simulink model "SC_LQR_simple_voltage_model"  (R2023a)
settings: Solver=VariableStepAuto  StartTime=0.0  StopTime=200  RelTol=1e-3
values from neighbouring files (symbols this model uses):
  A_model = [A11 zeros(3) A13 ... (first row only)    [LQR_state_space.m]
  B_model = [I^-1 I^-1 I^-1 ... (first row only)    [LQR_state_space.m]
  C_model = [eye(3) zeros(3) zeros(3) ... (first row only)    [LQR_state_space.m]
  D_model = [zeros(3) zeros(3) zeros(3) ... (first row only)    [LQR_state_space.m]
  I = 1e-7*[336109.715 0 0 ... (first row only)    [LQR_state_space.m]
  K1 = K(1:3,:)    [LQR_state_space.m]
  K2 = K(4:6,:)    [LQR_state_space.m]
  K3 = K(7:9,:)    [LQR_state_space.m]
  x0 = zeros(9,1)    [LQR_state_space.m]
undefined symbols (not defined in the file or in its folder): A, A_motor, B, B_motor, C_motor, D_motor, J, juliandate, K, Ke, Kt, La, n_cal, R_mgt, Ra, T_ext, T_max, T_max_mgt
libraries: matrix_library x15, slpidlib x15, simulink_extras x6, sharedutil x3, aerolibutil x2, vrlib x2, aerolibcubesatveh x1, aerolibgravity2 x1
(part 2 of 3)

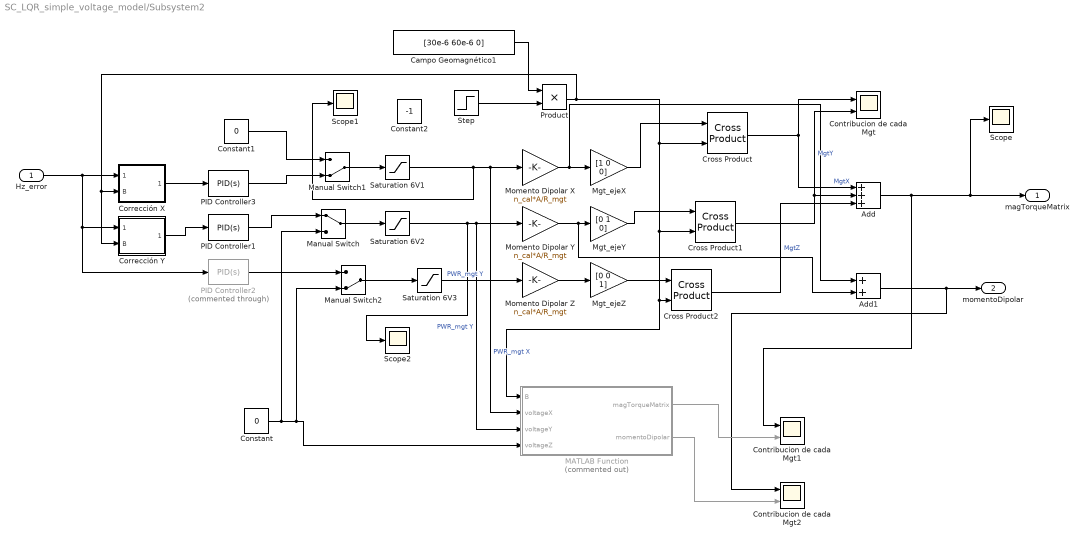
== system SC_LQR_simple_voltage_model/Subsystem2 ==
  Hz_error : Inport
  Add : Sum  Inputs=+++
  Add1 : Sum
  Campo Geomagnético1 : Constant  Value=[30e-6 60e-6 0]
  Constant : Constant  Value=0
  Constant1 : Constant  Value=0
  Constant2 : Constant  Value=-1
  Contribucion de cada Mgt : Scope  NumInputPorts=2
  Contribucion de cada Mgt1 : Scope  NumInputPorts=2
  Contribucion de cada Mgt2 : Scope  NumInputPorts=2
  Corrección X : MATLAB Function  TreatAsAtomicUnit=on
  Corrección Y : MATLAB Function  TreatAsAtomicUnit=on
  Cross Product : matrix_library/Cross Product
  Cross Product1 : matrix_library/Cross Product
  Cross Product2 : matrix_library/Cross Product
  MATLAB Function : MATLAB Function  Commented=on  TreatAsAtomicUnit=on
  Manual Switch : ManualSwitch
  Manual Switch1 : ManualSwitch  CurrentSetting=0
  Manual Switch2 : ManualSwitch  CurrentSetting=0
  Mgt_ejeX : Gain  Gain=[1 0 0]
  Mgt_ejeY : Gain  Gain=[0 1 0]
  Mgt_ejeZ : Gain  Gain=[0 0 1]
  Momento Dipolar X : Gain  Gain=n_cal*A/R_mgt
  Momento Dipolar Y : Gain  Gain=n_cal*A/R_mgt
  Momento Dipolar Z : Gain  Gain=n_cal*A/R_mgt
  PID Controller1 : slpidlib/PID Controller  Controller=PID  Form=Parallel  TimeDomain=Continuous-time  UseExternalTs=off  SampleTime=-1  IntegratorMethod=Forward Euler  FilterMethod=Forward Euler  ControllerParametersSource=internal  P=4500  I=800  UseKiTs=off  D=8000  N=100  UseFilter=on  TunerSelectOption=Transfer Function Based (PID Tuner App)  InitialConditionSource=internal  InitialConditionForIntegrator=0  InitialConditionForFilter=0  DifferentiatorICPrevScaledInput=0  ExternalReset=none  TrackingMode=off  Kt=1  LimitOutput=off  SatLimitsSource=internal  UpperSaturationLimit=1  LowerSaturationLimit=-1  LinearizeAsGain=on  AntiWindupMode=none  Kb=1  LimitIntegrator=off  UpperIntegratorSaturationLimit=inf  LowerIntegratorSaturationLimit=-inf  POutMin=[]  POutMax=[]  IOutMin=[]  IOutMax=[]  DOutMin=[]  DOutMax=[]  NOutMin=[]  NOutMax=[]  SumOutMin=[]  SumOutMax=[]  SaturationOutMin=[]  SaturationOutMax=[]  PParamMin=[]  PParamMax=[]  IParamMin=[]  IParamMax=[]  DParamMin=[]  DParamMax=[]  NParamMin=[]  NParamMax=[]  KbParamMin=[]  KbParamMax=[]  KtParamMin=[]  KtParamMax=[]  KbOutMin=[]  KbOutMax=[]  KtOutMin=[]  KtOutMax=[]  IntegratorOutMin=[]  IntegratorOutMax=[]  FilterOutMin=[]  FilterOutMax=[]  SumI1OutMin=[]  SumI1OutMax=[]  SumI2OutMin=[]  SumI2OutMax=[]  SumI3OutMin=[]  SumI3OutMax=[]  SumI4OutMin=[]  SumI4OutMax=[]  SumDOutMin=[]  SumDOutMax=[]  DifferentiatorOutMin=[]  DifferentiatorOutMax=[]  FilterDiffOutCoefMin=[]  FilterDiffOutCoefMax=[]  ReciprocalOutMin=[]  ReciprocalOutMax=[]  SumDenOutMin=[]  SumDenOutMax=[]  SumNumOutMin=[]  SumNumOutMax=[]  DivideOutMin=[]  DivideOutMax=[]  UdiffTsProdOutMin=[]  UdiffTsProdOutMax=[]  NTsProdOutMin=[]  NTsProdOutMax=[]  UintegralTsProdOutMin=[]  UintegralTsProdOutMax=[]  UngainTsProdOutMin=[]  UngainTsProdOutMax=[]  ClampingZeroOutDataTypeStr=Inherit: Inherit via back propagation  ClampingZeroOutMin=[]  ClampingZeroOutMax=[]  FilterDenConstantOutDataTypeStr=Inherit: Inherit via back propagation  FilterDenConstantOutMin=[]  FilterDenConstantOutMax=[]  PCopyOutDataTypeStr=Inherit: Inherit via back propagation  PCopyOutMin=[]  PCopyOutMax=[]  NCopyOutDataTypeStr=Inherit: Inherit via back propagation  NCopyOutMin=[]  NCopyOutMax=[]  IntegratorContinuousStateAttributes=''  IntegratorStateMustResolveToSignalObject=off  IntegratorRTWStateStorageClass=Auto  FilterContinuousStateAttributes=''  FilterStateMustResolveToSignalObject=off  FilterRTWStateStorageClass=Auto  ParallelPVariant=InternalParameters  IdealPVariant=Disabled  IVariant=InternalParameters  DVariant=InternalParameters  IntegratorVariant=Continuous  SatVariant=Disabled  AWVariant=Passthrough  PCopyVariant=Disabled  TRVariant=Disabled  FdbkBlocksVariant=Forward  IdealPFdbkVariant=Disabled  SatFdbkVariant=Disabled  DerivativeFilterVariant=ContFilter  NVariant=InternalParameters  NCopyVariant=Disabled  FilterICVariant=InternalICsFilter  IntegratorICVariant=InternalICs  ExternalResetVariant=Disabled  TRSumVariant=Passthrough  SumFdbkVariant=Disabled  SumVariant=Sum_PID  TsampFilterVariant=InternalTs  TsampNgainVariant=Passthrough  TsampIntegralVariant=Disabled_SignalSpec  ExternalSaturationOutDataTypeStr=Inherit: Same as second input
  PID Controller2 : slpidlib/PID Controller  Commented=through  Controller=PID  Form=Parallel  TimeDomain=Continuous-time  UseExternalTs=off  SampleTime=-1  IntegratorMethod=Forward Euler  FilterMethod=Forward Euler  ControllerParametersSource=internal  P=4500  I=800  UseKiTs=off  D=8000  N=100  UseFilter=on  TunerSelectOption=Transfer Function Based (PID Tuner App)  InitialConditionSource=internal  InitialConditionForIntegrator=0  InitialConditionForFilter=0  DifferentiatorICPrevScaledInput=0  ExternalReset=none  TrackingMode=off  Kt=1  LimitOutput=off  SatLimitsSource=internal  UpperSaturationLimit=1  LowerSaturationLimit=-1  LinearizeAsGain=on  AntiWindupMode=none  Kb=1  LimitIntegrator=off  UpperIntegratorSaturationLimit=inf  LowerIntegratorSaturationLimit=-inf  POutMin=[]  POutMax=[]  IOutMin=[]  IOutMax=[]  DOutMin=[]  DOutMax=[]  NOutMin=[]  NOutMax=[]  SumOutMin=[]  SumOutMax=[]  SaturationOutMin=[]  SaturationOutMax=[]  PParamMin=[]  PParamMax=[]  IParamMin=[]  IParamMax=[]  DParamMin=[]  DParamMax=[]  NParamMin=[]  NParamMax=[]  KbParamMin=[]  KbParamMax=[]  KtParamMin=[]  KtParamMax=[]  KbOutMin=[]  KbOutMax=[]  KtOutMin=[]  KtOutMax=[]  IntegratorOutMin=[]  IntegratorOutMax=[]  FilterOutMin=[]  FilterOutMax=[]  SumI1OutMin=[]  SumI1OutMax=[]  SumI2OutMin=[]  SumI2OutMax=[]  SumI3OutMin=[]  SumI3OutMax=[]  SumI4OutMin=[]  SumI4OutMax=[]  SumDOutMin=[]  SumDOutMax=[]  DifferentiatorOutMin=[]  DifferentiatorOutMax=[]  FilterDiffOutCoefMin=[]  FilterDiffOutCoefMax=[]  ReciprocalOutMin=[]  ReciprocalOutMax=[]  SumDenOutMin=[]  SumDenOutMax=[]  SumNumOutMin=[]  SumNumOutMax=[]  DivideOutMin=[]  DivideOutMax=[]  UdiffTsProdOutMin=[]  UdiffTsProdOutMax=[]  NTsProdOutMin=[]  NTsProdOutMax=[]  UintegralTsProdOutMin=[]  UintegralTsProdOutMax=[]  UngainTsProdOutMin=[]  UngainTsProdOutMax=[]  ClampingZeroOutDataTypeStr=Inherit: Inherit via back propagation  ClampingZeroOutMin=[]  ClampingZeroOutMax=[]  FilterDenConstantOutDataTypeStr=Inherit: Inherit via back propagation  FilterDenConstantOutMin=[]  FilterDenConstantOutMax=[]  PCopyOutDataTypeStr=Inherit: Inherit via back propagation  PCopyOutMin=[]  PCopyOutMax=[]  NCopyOutDataTypeStr=Inherit: Inherit via back propagation  NCopyOutMin=[]  NCopyOutMax=[]  IntegratorContinuousStateAttributes=''  IntegratorStateMustResolveToSignalObject=off  IntegratorRTWStateStorageClass=Auto  FilterContinuousStateAttributes=''  FilterStateMustResolveToSignalObject=off  FilterRTWStateStorageClass=Auto  ParallelPVariant=InternalParameters  IdealPVariant=Disabled  IVariant=InternalParameters  DVariant=InternalParameters  IntegratorVariant=Continuous  SatVariant=Disabled  AWVariant=Passthrough  PCopyVariant=Disabled  TRVariant=Disabled  FdbkBlocksVariant=Forward  IdealPFdbkVariant=Disabled  SatFdbkVariant=Disabled  DerivativeFilterVariant=ContFilter  NVariant=InternalParameters  NCopyVariant=Disabled  FilterICVariant=InternalICsFilter  IntegratorICVariant=InternalICs  ExternalResetVariant=Disabled  TRSumVariant=Passthrough  SumFdbkVariant=Disabled  SumVariant=Sum_PID  TsampFilterVariant=InternalTs  TsampNgainVariant=Passthrough  TsampIntegralVariant=Disabled_SignalSpec  ExternalSaturationOutDataTypeStr=Inherit: Same as second input
  PID Controller3 : slpidlib/PID Controller  Controller=PID  Form=Parallel  TimeDomain=Continuous-time  UseExternalTs=off  SampleTime=-1  IntegratorMethod=Forward Euler  FilterMethod=Forward Euler  ControllerParametersSource=internal  P=4500  I=800  UseKiTs=off  D=8000  N=100  UseFilter=on  TunerSelectOption=Transfer Function Based (PID Tuner App)  InitialConditionSource=internal  InitialConditionForIntegrator=0  InitialConditionForFilter=0  DifferentiatorICPrevScaledInput=0  ExternalReset=none  TrackingMode=off  Kt=1  LimitOutput=off  SatLimitsSource=internal  UpperSaturationLimit=1  LowerSaturationLimit=-1  LinearizeAsGain=on  AntiWindupMode=none  Kb=1  LimitIntegrator=off  UpperIntegratorSaturationLimit=inf  LowerIntegratorSaturationLimit=-inf  POutMin=[]  POutMax=[]  IOutMin=[]  IOutMax=[]  DOutMin=[]  DOutMax=[]  NOutMin=[]  NOutMax=[]  SumOutMin=[]  SumOutMax=[]  SaturationOutMin=[]  SaturationOutMax=[]  PParamMin=[]  PParamMax=[]  IParamMin=[]  IParamMax=[]  DParamMin=[]  DParamMax=[]  NParamMin=[]  NParamMax=[]  KbParamMin=[]  KbParamMax=[]  KtParamMin=[]  KtParamMax=[]  KbOutMin=[]  KbOutMax=[]  KtOutMin=[]  KtOutMax=[]  IntegratorOutMin=[]  IntegratorOutMax=[]  FilterOutMin=[]  FilterOutMax=[]  SumI1OutMin=[]  SumI1OutMax=[]  SumI2OutMin=[]  SumI2OutMax=[]  SumI3OutMin=[]  SumI3OutMax=[]  SumI4OutMin=[]  SumI4OutMax=[]  SumDOutMin=[]  SumDOutMax=[]  DifferentiatorOutMin=[]  DifferentiatorOutMax=[]  FilterDiffOutCoefMin=[]  FilterDiffOutCoefMax=[]  ReciprocalOutMin=[]  ReciprocalOutMax=[]  SumDenOutMin=[]  SumDenOutMax=[]  SumNumOutMin=[]  SumNumOutMax=[]  DivideOutMin=[]  DivideOutMax=[]  UdiffTsProdOutMin=[]  UdiffTsProdOutMax=[]  NTsProdOutMin=[]  NTsProdOutMax=[]  UintegralTsProdOutMin=[]  UintegralTsProdOutMax=[]  UngainTsProdOutMin=[]  UngainTsProdOutMax=[]  ClampingZeroOutDataTypeStr=Inherit: Inherit via back propagation  ClampingZeroOutMin=[]  ClampingZeroOutMax=[]  FilterDenConstantOutDataTypeStr=Inherit: Inherit via back propagation  FilterDenConstantOutMin=[]  FilterDenConstantOutMax=[]  PCopyOutDataTypeStr=Inherit: Inherit via back propagation  PCopyOutMin=[]  PCopyOutMax=[]  NCopyOutDataTypeStr=Inherit: Inherit via back propagation  NCopyOutMin=[]  NCopyOutMax=[]  IntegratorContinuousStateAttributes=''  IntegratorStateMustResolveToSignalObject=off  IntegratorRTWStateStorageClass=Auto  FilterContinuousStateAttributes=''  FilterStateMustResolveToSignalObject=off  FilterRTWStateStorageClass=Auto  ParallelPVariant=InternalParameters  IdealPVariant=Disabled  IVariant=InternalParameters  DVariant=InternalParameters  IntegratorVariant=Continuous  SatVariant=Disabled  AWVariant=Passthrough  PCopyVariant=Disabled  TRVariant=Disabled  FdbkBlocksVariant=Forward  IdealPFdbkVariant=Disabled  SatFdbkVariant=Disabled  DerivativeFilterVariant=ContFilter  NVariant=InternalParameters  NCopyVariant=Disabled  FilterICVariant=InternalICsFilter  IntegratorICVariant=InternalICs  ExternalResetVariant=Disabled  TRSumVariant=Passthrough  SumFdbkVariant=Disabled  SumVariant=Sum_PID  TsampFilterVariant=InternalTs  TsampNgainVariant=Passthrough  TsampIntegralVariant=Disabled_SignalSpec  ExternalSaturationOutDataTypeStr=Inherit: Same as second input
  Product : Product
  Saturation 6V1 : Saturate  UpperLimit=5  LowerLimit=-5
  Saturation 6V2 : Saturate  UpperLimit=5  LowerLimit=-5
  Saturation 6V3 : Saturate  UpperLimit=5  LowerLimit=-5
  Scope : Scope
  Scope1 : Scope
  Scope2 : Scope
  Step : Step  Time=0  After=-1  SampleTime=0
  magTorqueMatrix : Outport
  momentoDipolar : Outport  Port=2
  wires:
  Corrección Y/1(H_error) -> PID Controller1/1
  Corrección X/1(H_error) -> PID Controller3/1
  Step/1 -> Product/2
  Campo Geomagnético1/1 -> Product/1
  Cross Product2/1 -> Add/3  "MgtZ"
  Mgt_ejeZ/1 -> Cross Product2/1
  Momento Dipolar Z/1 -> Mgt_ejeZ/1
  Saturation 6V3/1 -> Momento Dipolar Z/1  "PWR_mgt Y"
  PID Controller2/1 -> Manual Switch2/1
  Manual Switch2/1 -> Saturation 6V3/1
  MATLAB Function/2(momentoDipolar) -> Contribucion de cada Mgt2/2
  Add1/1 -> momentoDipolar/1, Contribucion de cada Mgt2/1
  MATLAB Function/1(magTorqueMatrix) -> Contribucion de cada Mgt1/2
  Add/1 -> magTorqueMatrix/1, Scope/1, Contribucion de cada Mgt1/1
  Cross Product1/1 -> Add/2, Contribucion de cada Mgt/2  "MgtY"
  Mgt_ejeY/1 -> Cross Product1/1
  Momento Dipolar Y/1 -> Mgt_ejeY/1, Add1/2
  Saturation 6V2/1 -> Momento Dipolar Y/1, MATLAB Function/3(voltageY), Scope2/1  "PWR_mgt Y"
  Cross Product/1 -> Contribucion de cada Mgt/1, Add/1  "MgtX"
  Mgt_ejeX/1 -> Cross Product/1
  Momento Dipolar X/1 -> Mgt_ejeX/1, Add1/1
  Manual Switch1/1 -> Saturation 6V1/1
  Constant1/1 -> Manual Switch1/1
  Constant/1 -> Manual Switch/2, MATLAB Function/4(voltageZ), Manual Switch2/2
  PID Controller1/1 -> Manual Switch/1
  Manual Switch/1 -> Saturation 6V2/1
  Product/1 -> Cross Product/2, Cross Product1/2, Cross Product2/2, MATLAB Function/1(B), Corrección X/2(B), Corrección Y/2(B)
  Hz_error/1 -> Corrección X/1("H_error "), Corrección Y/1("H_error "), PID Controller2/1
  Saturation 6V1/1 -> Momento Dipolar X/1, MATLAB Function/2(voltageX), Scope1/1  "PWR_mgt X"
  PID Controller3/1 -> Manual Switch1/2

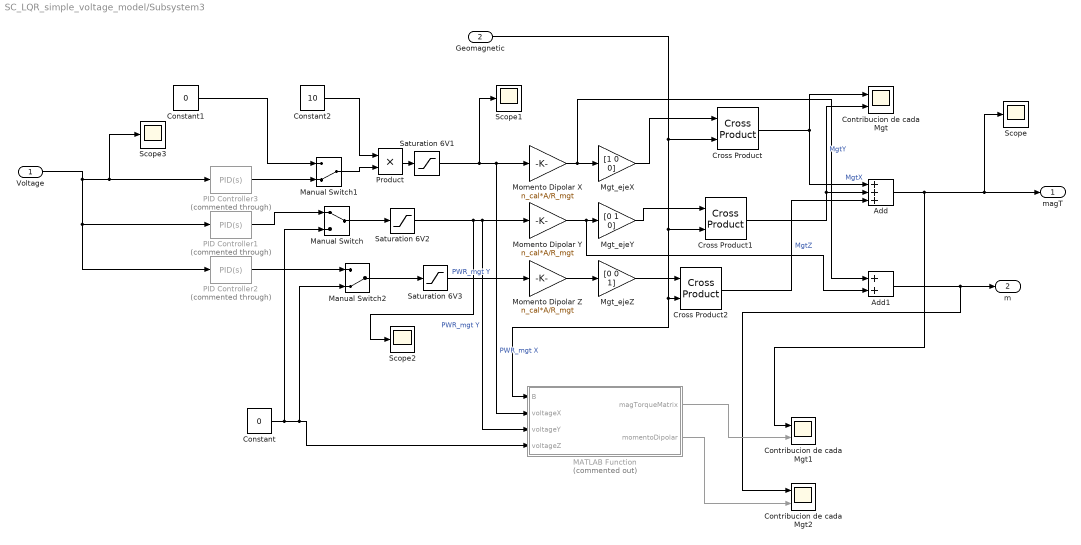
== system SC_LQR_simple_voltage_model/Subsystem3 ==
  Voltage : Inport
  Geomagnetic : Inport  Port=2
  Add : Sum  Inputs=+++
  Add1 : Sum
  Constant : Constant  Value=0
  Constant1 : Constant  Value=0
  Constant2 : Constant  Value=10
  Contribucion de cada Mgt : Scope  NumInputPorts=2
  Contribucion de cada Mgt1 : Scope  NumInputPorts=2
  Contribucion de cada Mgt2 : Scope  NumInputPorts=2
  Cross Product : matrix_library/Cross Product
  Cross Product1 : matrix_library/Cross Product
  Cross Product2 : matrix_library/Cross Product
  MATLAB Function : MATLAB Function  Commented=on  TreatAsAtomicUnit=on
  Manual Switch : ManualSwitch
  Manual Switch1 : ManualSwitch  CurrentSetting=0
  Manual Switch2 : ManualSwitch  CurrentSetting=0
  Mgt_ejeX : Gain  Gain=[1 0 0]
  Mgt_ejeY : Gain  Gain=[0 1 0]
  Mgt_ejeZ : Gain  Gain=[0 0 1]
  Momento Dipolar X : Gain  Gain=n_cal*A/R_mgt
  Momento Dipolar Y : Gain  Gain=n_cal*A/R_mgt
  Momento Dipolar Z : Gain  Gain=n_cal*A/R_mgt
  PID Controller1 : slpidlib/PID Controller  Commented=through  Controller=PID  Form=Parallel  TimeDomain=Continuous-time  UseExternalTs=off  SampleTime=-1  IntegratorMethod=Forward Euler  FilterMethod=Forward Euler  ControllerParametersSource=internal  P=4500  I=800  UseKiTs=off  D=8000  N=100  UseFilter=on  TunerSelectOption=Transfer Function Based (PID Tuner App)  InitialConditionSource=internal  InitialConditionForIntegrator=0  InitialConditionForFilter=0  DifferentiatorICPrevScaledInput=0  ExternalReset=none  TrackingMode=off  Kt=1  LimitOutput=off  SatLimitsSource=internal  UpperSaturationLimit=1  LowerSaturationLimit=-1  LinearizeAsGain=on  AntiWindupMode=none  Kb=1  LimitIntegrator=off  UpperIntegratorSaturationLimit=inf  LowerIntegratorSaturationLimit=-inf  POutMin=[]  POutMax=[]  IOutMin=[]  IOutMax=[]  DOutMin=[]  DOutMax=[]  NOutMin=[]  NOutMax=[]  SumOutMin=[]  SumOutMax=[]  SaturationOutMin=[]  SaturationOutMax=[]  PParamMin=[]  PParamMax=[]  IParamMin=[]  IParamMax=[]  DParamMin=[]  DParamMax=[]  NParamMin=[]  NParamMax=[]  KbParamMin=[]  KbParamMax=[]  KtParamMin=[]  KtParamMax=[]  KbOutMin=[]  KbOutMax=[]  KtOutMin=[]  KtOutMax=[]  IntegratorOutMin=[]  IntegratorOutMax=[]  FilterOutMin=[]  FilterOutMax=[]  SumI1OutMin=[]  SumI1OutMax=[]  SumI2OutMin=[]  SumI2OutMax=[]  SumI3OutMin=[]  SumI3OutMax=[]  SumI4OutMin=[]  SumI4OutMax=[]  SumDOutMin=[]  SumDOutMax=[]  DifferentiatorOutMin=[]  DifferentiatorOutMax=[]  FilterDiffOutCoefMin=[]  FilterDiffOutCoefMax=[]  ReciprocalOutMin=[]  ReciprocalOutMax=[]  SumDenOutMin=[]  SumDenOutMax=[]  SumNumOutMin=[]  SumNumOutMax=[]  DivideOutMin=[]  DivideOutMax=[]  UdiffTsProdOutMin=[]  UdiffTsProdOutMax=[]  NTsProdOutMin=[]  NTsProdOutMax=[]  UintegralTsProdOutMin=[]  UintegralTsProdOutMax=[]  UngainTsProdOutMin=[]  UngainTsProdOutMax=[]  ClampingZeroOutDataTypeStr=Inherit: Inherit via back propagation  ClampingZeroOutMin=[]  ClampingZeroOutMax=[]  FilterDenConstantOutDataTypeStr=Inherit: Inherit via back propagation  FilterDenConstantOutMin=[]  FilterDenConstantOutMax=[]  PCopyOutDataTypeStr=Inherit: Inherit via back propagation  PCopyOutMin=[]  PCopyOutMax=[]  NCopyOutDataTypeStr=Inherit: Inherit via back propagation  NCopyOutMin=[]  NCopyOutMax=[]  IntegratorContinuousStateAttributes=''  IntegratorStateMustResolveToSignalObject=off  IntegratorRTWStateStorageClass=Auto  FilterContinuousStateAttributes=''  FilterStateMustResolveToSignalObject=off  FilterRTWStateStorageClass=Auto  ParallelPVariant=InternalParameters  IdealPVariant=Disabled  IVariant=InternalParameters  DVariant=InternalParameters  IntegratorVariant=Continuous  SatVariant=Disabled  AWVariant=Passthrough  PCopyVariant=Disabled  TRVariant=Disabled  FdbkBlocksVariant=Forward  IdealPFdbkVariant=Disabled  SatFdbkVariant=Disabled  DerivativeFilterVariant=ContFilter  NVariant=InternalParameters  NCopyVariant=Disabled  FilterICVariant=InternalICsFilter  IntegratorICVariant=InternalICs  ExternalResetVariant=Disabled  TRSumVariant=Passthrough  SumFdbkVariant=Disabled  SumVariant=Sum_PID  TsampFilterVariant=InternalTs  TsampNgainVariant=Passthrough  TsampIntegralVariant=Disabled_SignalSpec  ExternalSaturationOutDataTypeStr=Inherit: Same as second input
  PID Controller2 : slpidlib/PID Controller  Commented=through  Controller=PID  Form=Parallel  TimeDomain=Continuous-time  UseExternalTs=off  SampleTime=-1  IntegratorMethod=Forward Euler  FilterMethod=Forward Euler  ControllerParametersSource=internal  P=4500  I=800  UseKiTs=off  D=8000  N=100  UseFilter=on  TunerSelectOption=Transfer Function Based (PID Tuner App)  InitialConditionSource=internal  InitialConditionForIntegrator=0  InitialConditionForFilter=0  DifferentiatorICPrevScaledInput=0  ExternalReset=none  TrackingMode=off  Kt=1  LimitOutput=off  SatLimitsSource=internal  UpperSaturationLimit=1  LowerSaturationLimit=-1  LinearizeAsGain=on  AntiWindupMode=none  Kb=1  LimitIntegrator=off  UpperIntegratorSaturationLimit=inf  LowerIntegratorSaturationLimit=-inf  POutMin=[]  POutMax=[]  IOutMin=[]  IOutMax=[]  DOutMin=[]  DOutMax=[]  NOutMin=[]  NOutMax=[]  SumOutMin=[]  SumOutMax=[]  SaturationOutMin=[]  SaturationOutMax=[]  PParamMin=[]  PParamMax=[]  IParamMin=[]  IParamMax=[]  DParamMin=[]  DParamMax=[]  NParamMin=[]  NParamMax=[]  KbParamMin=[]  KbParamMax=[]  KtParamMin=[]  KtParamMax=[]  KbOutMin=[]  KbOutMax=[]  KtOutMin=[]  KtOutMax=[]  IntegratorOutMin=[]  IntegratorOutMax=[]  FilterOutMin=[]  FilterOutMax=[]  SumI1OutMin=[]  SumI1OutMax=[]  SumI2OutMin=[]  SumI2OutMax=[]  SumI3OutMin=[]  SumI3OutMax=[]  SumI4OutMin=[]  SumI4OutMax=[]  SumDOutMin=[]  SumDOutMax=[]  DifferentiatorOutMin=[]  DifferentiatorOutMax=[]  FilterDiffOutCoefMin=[]  FilterDiffOutCoefMax=[]  ReciprocalOutMin=[]  ReciprocalOutMax=[]  SumDenOutMin=[]  SumDenOutMax=[]  SumNumOutMin=[]  SumNumOutMax=[]  DivideOutMin=[]  DivideOutMax=[]  UdiffTsProdOutMin=[]  UdiffTsProdOutMax=[]  NTsProdOutMin=[]  NTsProdOutMax=[]  UintegralTsProdOutMin=[]  UintegralTsProdOutMax=[]  UngainTsProdOutMin=[]  UngainTsProdOutMax=[]  ClampingZeroOutDataTypeStr=Inherit: Inherit via back propagation  ClampingZeroOutMin=[]  ClampingZeroOutMax=[]  FilterDenConstantOutDataTypeStr=Inherit: Inherit via back propagation  FilterDenConstantOutMin=[]  FilterDenConstantOutMax=[]  PCopyOutDataTypeStr=Inherit: Inherit via back propagation  PCopyOutMin=[]  PCopyOutMax=[]  NCopyOutDataTypeStr=Inherit: Inherit via back propagation  NCopyOutMin=[]  NCopyOutMax=[]  IntegratorContinuousStateAttributes=''  IntegratorStateMustResolveToSignalObject=off  IntegratorRTWStateStorageClass=Auto  FilterContinuousStateAttributes=''  FilterStateMustResolveToSignalObject=off  FilterRTWStateStorageClass=Auto  ParallelPVariant=InternalParameters  IdealPVariant=Disabled  IVariant=InternalParameters  DVariant=InternalParameters  IntegratorVariant=Continuous  SatVariant=Disabled  AWVariant=Passthrough  PCopyVariant=Disabled  TRVariant=Disabled  FdbkBlocksVariant=Forward  IdealPFdbkVariant=Disabled  SatFdbkVariant=Disabled  DerivativeFilterVariant=ContFilter  NVariant=InternalParameters  NCopyVariant=Disabled  FilterICVariant=InternalICsFilter  IntegratorICVariant=InternalICs  ExternalResetVariant=Disabled  TRSumVariant=Passthrough  SumFdbkVariant=Disabled  SumVariant=Sum_PID  TsampFilterVariant=InternalTs  TsampNgainVariant=Passthrough  TsampIntegralVariant=Disabled_SignalSpec  ExternalSaturationOutDataTypeStr=Inherit: Same as second input
  PID Controller3 : slpidlib/PID Controller  Commented=through  Controller=PID  Form=Parallel  TimeDomain=Continuous-time  UseExternalTs=off  SampleTime=-1  IntegratorMethod=Forward Euler  FilterMethod=Forward Euler  ControllerParametersSource=internal  P=4500  I=800  UseKiTs=off  D=8000  N=100  UseFilter=on  TunerSelectOption=Transfer Function Based (PID Tuner App)  InitialConditionSource=internal  InitialConditionForIntegrator=0  InitialConditionForFilter=0  DifferentiatorICPrevScaledInput=0  ExternalReset=none  TrackingMode=off  Kt=1  LimitOutput=off  SatLimitsSource=internal  UpperSaturationLimit=1  LowerSaturationLimit=-1  LinearizeAsGain=on  AntiWindupMode=none  Kb=1  LimitIntegrator=off  UpperIntegratorSaturationLimit=inf  LowerIntegratorSaturationLimit=-inf  POutMin=[]  POutMax=[]  IOutMin=[]  IOutMax=[]  DOutMin=[]  DOutMax=[]  NOutMin=[]  NOutMax=[]  SumOutMin=[]  SumOutMax=[]  SaturationOutMin=[]  SaturationOutMax=[]  PParamMin=[]  PParamMax=[]  IParamMin=[]  IParamMax=[]  DParamMin=[]  DParamMax=[]  NParamMin=[]  NParamMax=[]  KbParamMin=[]  KbParamMax=[]  KtParamMin=[]  KtParamMax=[]  KbOutMin=[]  KbOutMax=[]  KtOutMin=[]  KtOutMax=[]  IntegratorOutMin=[]  IntegratorOutMax=[]  FilterOutMin=[]  FilterOutMax=[]  SumI1OutMin=[]  SumI1OutMax=[]  SumI2OutMin=[]  SumI2OutMax=[]  SumI3OutMin=[]  SumI3OutMax=[]  SumI4OutMin=[]  SumI4OutMax=[]  SumDOutMin=[]  SumDOutMax=[]  DifferentiatorOutMin=[]  DifferentiatorOutMax=[]  FilterDiffOutCoefMin=[]  FilterDiffOutCoefMax=[]  ReciprocalOutMin=[]  ReciprocalOutMax=[]  SumDenOutMin=[]  SumDenOutMax=[]  SumNumOutMin=[]  SumNumOutMax=[]  DivideOutMin=[]  DivideOutMax=[]  UdiffTsProdOutMin=[]  UdiffTsProdOutMax=[]  NTsProdOutMin=[]  NTsProdOutMax=[]  UintegralTsProdOutMin=[]  UintegralTsProdOutMax=[]  UngainTsProdOutMin=[]  UngainTsProdOutMax=[]  ClampingZeroOutDataTypeStr=Inherit: Inherit via back propagation  ClampingZeroOutMin=[]  ClampingZeroOutMax=[]  FilterDenConstantOutDataTypeStr=Inherit: Inherit via back propagation  FilterDenConstantOutMin=[]  FilterDenConstantOutMax=[]  PCopyOutDataTypeStr=Inherit: Inherit via back propagation  PCopyOutMin=[]  PCopyOutMax=[]  NCopyOutDataTypeStr=Inherit: Inherit via back propagation  NCopyOutMin=[]  NCopyOutMax=[]  IntegratorContinuousStateAttributes=''  IntegratorStateMustResolveToSignalObject=off  IntegratorRTWStateStorageClass=Auto  FilterContinuousStateAttributes=''  FilterStateMustResolveToSignalObject=off  FilterRTWStateStorageClass=Auto  ParallelPVariant=InternalParameters  IdealPVariant=Disabled  IVariant=InternalParameters  DVariant=InternalParameters  IntegratorVariant=Continuous  SatVariant=Disabled  AWVariant=Passthrough  PCopyVariant=Disabled  TRVariant=Disabled  FdbkBlocksVariant=Forward  IdealPFdbkVariant=Disabled  SatFdbkVariant=Disabled  DerivativeFilterVariant=ContFilter  NVariant=InternalParameters  NCopyVariant=Disabled  FilterICVariant=InternalICsFilter  IntegratorICVariant=InternalICs  ExternalResetVariant=Disabled  TRSumVariant=Passthrough  SumFdbkVariant=Disabled  SumVariant=Sum_PID  TsampFilterVariant=InternalTs  TsampNgainVariant=Passthrough  TsampIntegralVariant=Disabled_SignalSpec  ExternalSaturationOutDataTypeStr=Inherit: Same as second input
  Product : Product
  Saturation 6V1 : Saturate  UpperLimit=5  LowerLimit=-5
  Saturation 6V2 : Saturate  UpperLimit=5  LowerLimit=-5
  Saturation 6V3 : Saturate  UpperLimit=5  LowerLimit=-5
  Scope{,1..3} (4 alike) : Scope
  magT : Outport
  m : Outport  Port=2
  wires:
  Voltage/1 -> PID Controller2/1, PID Controller1/1, Scope3/1, PID Controller3/1
  Cross Product2/1 -> Add/3  "MgtZ"
  Mgt_ejeZ/1 -> Cross Product2/1
  Momento Dipolar Z/1 -> Mgt_ejeZ/1
  Saturation 6V3/1 -> Momento Dipolar Z/1  "PWR_mgt Y"
  PID Controller2/1 -> Manual Switch2/1
  Manual Switch2/1 -> Saturation 6V3/1
  MATLAB Function/2(momentoDipolar) -> Contribucion de cada Mgt2/2
  Add1/1 -> m/1, Contribucion de cada Mgt2/1
  MATLAB Function/1(magTorqueMatrix) -> Contribucion de cada Mgt1/2
  Add/1 -> magT/1, Scope/1, Contribucion de cada Mgt1/1
  Cross Product1/1 -> Add/2, Contribucion de cada Mgt/2  "MgtY"
  Mgt_ejeY/1 -> Cross Product1/1
  Momento Dipolar Y/1 -> Mgt_ejeY/1, Add1/2
  Saturation 6V2/1 -> Momento Dipolar Y/1, MATLAB Function/3(voltageY), Scope2/1  "PWR_mgt Y"
  Cross Product/1 -> Contribucion de cada Mgt/1, Add/1  "MgtX"
  Mgt_ejeX/1 -> Cross Product/1
  Momento Dipolar X/1 -> Mgt_ejeX/1, Add1/1
  Constant1/1 -> Manual Switch1/1
  Constant/1 -> Manual Switch/2, MATLAB Function/4(voltageZ), Manual Switch2/2
  PID Controller1/1 -> Manual Switch/1
  Manual Switch/1 -> Saturation 6V2/1
  Geomagnetic/1 -> Cross Product/2, Cross Product1/2, Cross Product2/2, MATLAB Function/1(B)
  Saturation 6V1/1 -> Momento Dipolar X/1, MATLAB Function/2(voltageX), Scope1/1  "PWR_mgt X"
  PID Controller3/1 -> Manual Switch1/2
  Product/1 -> Saturation 6V1/1
  Manual Switch1/1 -> Product/2
  Constant2/1 -> Product/1

== system SC_LQR_simple_voltage_model/Subsystem4 ==
  euler angles : Inport
  Constant : Constant  Value=2019
  CubeSat Vehicle : aerolibcubesatveh/CubeSat Vehicle (Nadir Pointing)  sim_t0=juliandate(2019, 1, 4, 12, 0, 0)  method=Keplerian Orbital Elements  epoch=juliandate(2020, 1, 1, 12, 0, 0)  a=6786233.13  ecc=0.0010537  incl=51.7519  omega=95.2562  argp=93.4872  nu=302.9234  truelon=0  arglat=0  lonper=0  r_eci=[0 0 0]  v_eci=[0 0 0]  r_ecef=[0 0 0]  v_ecef=[0 0 0]  lla=[0 0 0]  v_ned=[0 0 0]  euler=[0 0 0]  pqr=[0 0 -0.05168]  pointingMode=Earth (Nadir) Pointing  firstAlignExt=Dialog  firstAlign=[0 0 1]  secondAlignExt=Dialog  secondAlign=[0 1 0]  constraintCoord=ECI Axes  firstRefExt=Dialog  firstRef=[1 0 0]  secondRefExt=Dialog  secondRef=[0 0 1]  missionRTSource=Dialog  missionRT=6*60*60  missionGS=[42, -71]  missionTOICheck=on  missionTOI=[]  missionEta=55
      settings: AttributesFormatString=%<pointingMode>
  Demux4 : Demux  Outputs=2
  ECEF Position to LLA : ECEF2LLA
  Environment Models : Subsystem
      mask Display:
      | port_label('input', 1, 'X_{ECEF}','texmode','on')
      | port_label('input', 2, 'V_{ECEF}','texmode','on')
      | port_label('output', 1, 'A_{ECEF}','texmode','on')
  MATLAB Function : MATLAB Function  TreatAsAtomicUnit=on
  Scope8 : Scope
  World Magnetic Model : aerolibgravity2/World Magnetic Model  model=WMM2015 V2 (2015-2020)  customFile='WMM2020.COF'  units=Metric (MKS)  time_in=on  month=January  day=1  year=2020  action=Error  h_out=on  dec_out=on  inc_out=on  ti_out=on
  nT to T : Gain  Gain=1e-9
  B : Outport
  wires:
  ECEF Position to LLA/2 -> World Magnetic Model/1
  Environment Models/1(a_ff) -> CubeSat Vehicle/1
  Constant/1 -> World Magnetic Model/4
  nT to T/1 -> MATLAB Function/1(NEDMagnetic), Scope8/1
  World Magnetic Model/1 -> nT to T/1
  CubeSat Vehicle/1 -> ECEF Position to LLA/1, Environment Models/1(x_ff)
  Demux4/2 -> World Magnetic Model/3
  euler angles/1 -> MATLAB Function/2(RPY)
  CubeSat Vehicle/2 -> Environment Models/2(v_ff)
  MATLAB Function/1(RPY_Magnetic) -> B/1
  ECEF Position to LLA/1 -> Demux4/1
  Demux4/1 -> World Magnetic Model/2

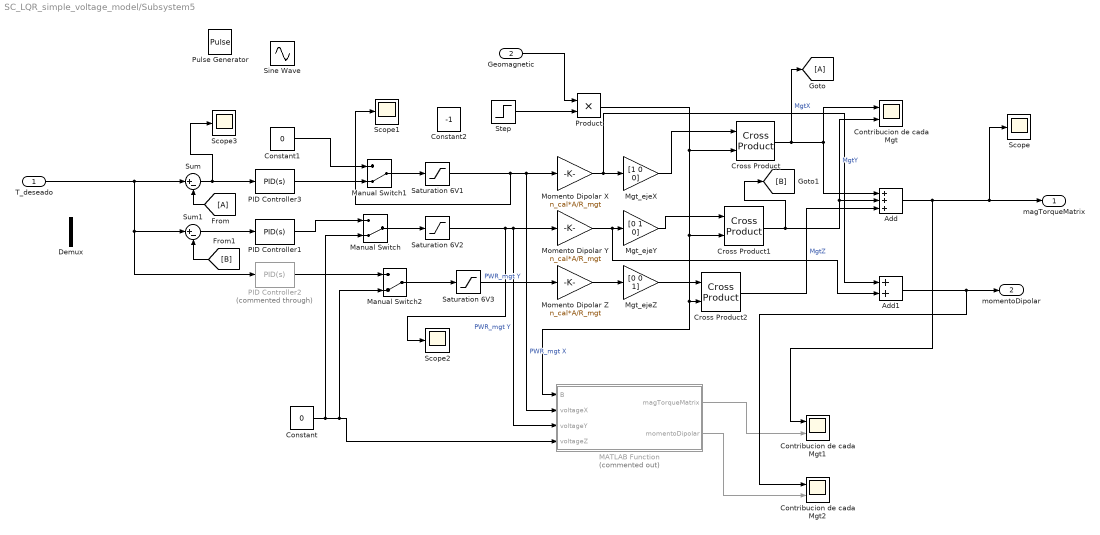
== system SC_LQR_simple_voltage_model/Subsystem5 ==
  T_deseado : Inport
  Geomagnetic : Inport  Port=2
  Add : Sum  Inputs=+++
  Add1 : Sum
  Constant : Constant  Value=0
  Constant1 : Constant  Value=0
  Constant2 : Constant  Value=-1
  Contribucion de cada Mgt : Scope  NumInputPorts=2
  Contribucion de cada Mgt1 : Scope  NumInputPorts=2
  Contribucion de cada Mgt2 : Scope  NumInputPorts=2
  Cross Product : matrix_library/Cross Product
  Cross Product1 : matrix_library/Cross Product
  Cross Product2 : matrix_library/Cross Product
  Demux : Demux  Outputs=2
  From : From
  Goto : Goto
  MATLAB Function : MATLAB Function  Commented=on  TreatAsAtomicUnit=on
  Manual Switch : ManualSwitch  CurrentSetting=0
  Manual Switch1 : ManualSwitch  CurrentSetting=0
  Manual Switch2 : ManualSwitch  CurrentSetting=0
  Mgt_ejeX : Gain  Gain=[1 0 0]
  Mgt_ejeY : Gain  Gain=[0 1 0]
  Mgt_ejeZ : Gain  Gain=[0 0 1]
  Momento Dipolar X : Gain  Gain=n_cal*A/R_mgt
  Momento Dipolar Y : Gain  Gain=n_cal*A/R_mgt
  Momento Dipolar Z : Gain  Gain=n_cal*A/R_mgt
  PID Controller1 : slpidlib/PID Controller  Controller=PID  Form=Parallel  TimeDomain=Continuous-time  UseExternalTs=off  SampleTime=-1  IntegratorMethod=Forward Euler  FilterMethod=Forward Euler  ControllerParametersSource=internal  P=4500  I=800  UseKiTs=off  D=8000  N=100  UseFilter=on  TunerSelectOption=Transfer Function Based (PID Tuner App)  InitialConditionSource=internal  InitialConditionForIntegrator=0  InitialConditionForFilter=0  DifferentiatorICPrevScaledInput=0  ExternalReset=none  TrackingMode=off  Kt=1  LimitOutput=off  SatLimitsSource=internal  UpperSaturationLimit=1  LowerSaturationLimit=-1  LinearizeAsGain=on  AntiWindupMode=none  Kb=1  LimitIntegrator=off  UpperIntegratorSaturationLimit=inf  LowerIntegratorSaturationLimit=-inf  POutMin=[]  POutMax=[]  IOutMin=[]  IOutMax=[]  DOutMin=[]  DOutMax=[]  NOutMin=[]  NOutMax=[]  SumOutMin=[]  SumOutMax=[]  SaturationOutMin=[]  SaturationOutMax=[]  PParamMin=[]  PParamMax=[]  IParamMin=[]  IParamMax=[]  DParamMin=[]  DParamMax=[]  NParamMin=[]  NParamMax=[]  KbParamMin=[]  KbParamMax=[]  KtParamMin=[]  KtParamMax=[]  KbOutMin=[]  KbOutMax=[]  KtOutMin=[]  KtOutMax=[]  IntegratorOutMin=[]  IntegratorOutMax=[]  FilterOutMin=[]  FilterOutMax=[]  SumI1OutMin=[]  SumI1OutMax=[]  SumI2OutMin=[]  SumI2OutMax=[]  SumI3OutMin=[]  SumI3OutMax=[]  SumI4OutMin=[]  SumI4OutMax=[]  SumDOutMin=[]  SumDOutMax=[]  DifferentiatorOutMin=[]  DifferentiatorOutMax=[]  FilterDiffOutCoefMin=[]  FilterDiffOutCoefMax=[]  ReciprocalOutMin=[]  ReciprocalOutMax=[]  SumDenOutMin=[]  SumDenOutMax=[]  SumNumOutMin=[]  SumNumOutMax=[]  DivideOutMin=[]  DivideOutMax=[]  UdiffTsProdOutMin=[]  UdiffTsProdOutMax=[]  NTsProdOutMin=[]  NTsProdOutMax=[]  UintegralTsProdOutMin=[]  UintegralTsProdOutMax=[]  UngainTsProdOutMin=[]  UngainTsProdOutMax=[]  ClampingZeroOutDataTypeStr=Inherit: Inherit via back propagation  ClampingZeroOutMin=[]  ClampingZeroOutMax=[]  FilterDenConstantOutDataTypeStr=Inherit: Inherit via back propagation  FilterDenConstantOutMin=[]  FilterDenConstantOutMax=[]  PCopyOutDataTypeStr=Inherit: Inherit via back propagation  PCopyOutMin=[]  PCopyOutMax=[]  NCopyOutDataTypeStr=Inherit: Inherit via back propagation  NCopyOutMin=[]  NCopyOutMax=[]  IntegratorContinuousStateAttributes=''  IntegratorStateMustResolveToSignalObject=off  IntegratorRTWStateStorageClass=Auto  FilterContinuousStateAttributes=''  FilterStateMustResolveToSignalObject=off  FilterRTWStateStorageClass=Auto  ParallelPVariant=InternalParameters  IdealPVariant=Disabled  IVariant=InternalParameters  DVariant=InternalParameters  IntegratorVariant=Continuous  SatVariant=Disabled  AWVariant=Passthrough  PCopyVariant=Disabled  TRVariant=Disabled  FdbkBlocksVariant=Forward  IdealPFdbkVariant=Disabled  SatFdbkVariant=Disabled  DerivativeFilterVariant=ContFilter  NVariant=InternalParameters  NCopyVariant=Disabled  FilterICVariant=InternalICsFilter  IntegratorICVariant=InternalICs  ExternalResetVariant=Disabled  TRSumVariant=Passthrough  SumFdbkVariant=Disabled  SumVariant=Sum_PID  TsampFilterVariant=InternalTs  TsampNgainVariant=Passthrough  TsampIntegralVariant=Disabled_SignalSpec  ExternalSaturationOutDataTypeStr=Inherit: Same as second input
  PID Controller2 : slpidlib/PID Controller  Commented=through  Controller=PID  Form=Parallel  TimeDomain=Continuous-time  UseExternalTs=off  SampleTime=-1  IntegratorMethod=Forward Euler  FilterMethod=Forward Euler  ControllerParametersSource=internal  P=4500  I=800  UseKiTs=off  D=8000  N=100  UseFilter=on  TunerSelectOption=Transfer Function Based (PID Tuner App)  InitialConditionSource=internal  InitialConditionForIntegrator=0  InitialConditionForFilter=0  DifferentiatorICPrevScaledInput=0  ExternalReset=none  TrackingMode=off  Kt=1  LimitOutput=off  SatLimitsSource=internal  UpperSaturationLimit=1  LowerSaturationLimit=-1  LinearizeAsGain=on  AntiWindupMode=none  Kb=1  LimitIntegrator=off  UpperIntegratorSaturationLimit=inf  LowerIntegratorSaturationLimit=-inf  POutMin=[]  POutMax=[]  IOutMin=[]  IOutMax=[]  DOutMin=[]  DOutMax=[]  NOutMin=[]  NOutMax=[]  SumOutMin=[]  SumOutMax=[]  SaturationOutMin=[]  SaturationOutMax=[]  PParamMin=[]  PParamMax=[]  IParamMin=[]  IParamMax=[]  DParamMin=[]  DParamMax=[]  NParamMin=[]  NParamMax=[]  KbParamMin=[]  KbParamMax=[]  KtParamMin=[]  KtParamMax=[]  KbOutMin=[]  KbOutMax=[]  KtOutMin=[]  KtOutMax=[]  IntegratorOutMin=[]  IntegratorOutMax=[]  FilterOutMin=[]  FilterOutMax=[]  SumI1OutMin=[]  SumI1OutMax=[]  SumI2OutMin=[]  SumI2OutMax=[]  SumI3OutMin=[]  SumI3OutMax=[]  SumI4OutMin=[]  SumI4OutMax=[]  SumDOutMin=[]  SumDOutMax=[]  DifferentiatorOutMin=[]  DifferentiatorOutMax=[]  FilterDiffOutCoefMin=[]  FilterDiffOutCoefMax=[]  ReciprocalOutMin=[]  ReciprocalOutMax=[]  SumDenOutMin=[]  SumDenOutMax=[]  SumNumOutMin=[]  SumNumOutMax=[]  DivideOutMin=[]  DivideOutMax=[]  UdiffTsProdOutMin=[]  UdiffTsProdOutMax=[]  NTsProdOutMin=[]  NTsProdOutMax=[]  UintegralTsProdOutMin=[]  UintegralTsProdOutMax=[]  UngainTsProdOutMin=[]  UngainTsProdOutMax=[]  ClampingZeroOutDataTypeStr=Inherit: Inherit via back propagation  ClampingZeroOutMin=[]  ClampingZeroOutMax=[]  FilterDenConstantOutDataTypeStr=Inherit: Inherit via back propagation  FilterDenConstantOutMin=[]  FilterDenConstantOutMax=[]  PCopyOutDataTypeStr=Inherit: Inherit via back propagation  PCopyOutMin=[]  PCopyOutMax=[]  NCopyOutDataTypeStr=Inherit: Inherit via back propagation  NCopyOutMin=[]  NCopyOutMax=[]  IntegratorContinuousStateAttributes=''  IntegratorStateMustResolveToSignalObject=off  IntegratorRTWStateStorageClass=Auto  FilterContinuousStateAttributes=''  FilterStateMustResolveToSignalObject=off  FilterRTWStateStorageClass=Auto  ParallelPVariant=InternalParameters  IdealPVariant=Disabled  IVariant=InternalParameters  DVariant=InternalParameters  IntegratorVariant=Continuous  SatVariant=Disabled  AWVariant=Passthrough  PCopyVariant=Disabled  TRVariant=Disabled  FdbkBlocksVariant=Forward  IdealPFdbkVariant=Disabled  SatFdbkVariant=Disabled  DerivativeFilterVariant=ContFilter  NVariant=InternalParameters  NCopyVariant=Disabled  FilterICVariant=InternalICsFilter  IntegratorICVariant=InternalICs  ExternalResetVariant=Disabled  TRSumVariant=Passthrough  SumFdbkVariant=Disabled  SumVariant=Sum_PID  TsampFilterVariant=InternalTs  TsampNgainVariant=Passthrough  TsampIntegralVariant=Disabled_SignalSpec  ExternalSaturationOutDataTypeStr=Inherit: Same as second input
  PID Controller3 : slpidlib/PID Controller  Controller=PID  Form=Parallel  TimeDomain=Continuous-time  UseExternalTs=off  SampleTime=-1  IntegratorMethod=Forward Euler  FilterMethod=Forward Euler  ControllerParametersSource=internal  P=4500  I=800  UseKiTs=off  D=8000  N=100  UseFilter=on  TunerSelectOption=Transfer Function Based (PID Tuner App)  InitialConditionSource=internal  InitialConditionForIntegrator=0  InitialConditionForFilter=0  DifferentiatorICPrevScaledInput=0  ExternalReset=none  TrackingMode=off  Kt=1  LimitOutput=off  SatLimitsSource=internal  UpperSaturationLimit=1  LowerSaturationLimit=-1  LinearizeAsGain=on  AntiWindupMode=none  Kb=1  LimitIntegrator=off  UpperIntegratorSaturationLimit=inf  LowerIntegratorSaturationLimit=-inf  POutMin=[]  POutMax=[]  IOutMin=[]  IOutMax=[]  DOutMin=[]  DOutMax=[]  NOutMin=[]  NOutMax=[]  SumOutMin=[]  SumOutMax=[]  SaturationOutMin=[]  SaturationOutMax=[]  PParamMin=[]  PParamMax=[]  IParamMin=[]  IParamMax=[]  DParamMin=[]  DParamMax=[]  NParamMin=[]  NParamMax=[]  KbParamMin=[]  KbParamMax=[]  KtParamMin=[]  KtParamMax=[]  KbOutMin=[]  KbOutMax=[]  KtOutMin=[]  KtOutMax=[]  IntegratorOutMin=[]  IntegratorOutMax=[]  FilterOutMin=[]  FilterOutMax=[]  SumI1OutMin=[]  SumI1OutMax=[]  SumI2OutMin=[]  SumI2OutMax=[]  SumI3OutMin=[]  SumI3OutMax=[]  SumI4OutMin=[]  SumI4OutMax=[]  SumDOutMin=[]  SumDOutMax=[]  DifferentiatorOutMin=[]  DifferentiatorOutMax=[]  FilterDiffOutCoefMin=[]  FilterDiffOutCoefMax=[]  ReciprocalOutMin=[]  ReciprocalOutMax=[]  SumDenOutMin=[]  SumDenOutMax=[]  SumNumOutMin=[]  SumNumOutMax=[]  DivideOutMin=[]  DivideOutMax=[]  UdiffTsProdOutMin=[]  UdiffTsProdOutMax=[]  NTsProdOutMin=[]  NTsProdOutMax=[]  UintegralTsProdOutMin=[]  UintegralTsProdOutMax=[]  UngainTsProdOutMin=[]  UngainTsProdOutMax=[]  ClampingZeroOutDataTypeStr=Inherit: Inherit via back propagation  ClampingZeroOutMin=[]  ClampingZeroOutMax=[]  FilterDenConstantOutDataTypeStr=Inherit: Inherit via back propagation  FilterDenConstantOutMin=[]  FilterDenConstantOutMax=[]  PCopyOutDataTypeStr=Inherit: Inherit via back propagation  PCopyOutMin=[]  PCopyOutMax=[]  NCopyOutDataTypeStr=Inherit: Inherit via back propagation  NCopyOutMin=[]  NCopyOutMax=[]  IntegratorContinuousStateAttributes=''  IntegratorStateMustResolveToSignalObject=off  IntegratorRTWStateStorageClass=Auto  FilterContinuousStateAttributes=''  FilterStateMustResolveToSignalObject=off  FilterRTWStateStorageClass=Auto  ParallelPVariant=InternalParameters  IdealPVariant=Disabled  IVariant=InternalParameters  DVariant=InternalParameters  IntegratorVariant=Continuous  SatVariant=Disabled  AWVariant=Passthrough  PCopyVariant=Disabled  TRVariant=Disabled  FdbkBlocksVariant=Forward  IdealPFdbkVariant=Disabled  SatFdbkVariant=Disabled  DerivativeFilterVariant=ContFilter  NVariant=InternalParameters  NCopyVariant=Disabled  FilterICVariant=InternalICsFilter  IntegratorICVariant=InternalICs  ExternalResetVariant=Disabled  TRSumVariant=Passthrough  SumFdbkVariant=Disabled  SumVariant=Sum_PID  TsampFilterVariant=InternalTs  TsampNgainVariant=Passthrough  TsampIntegralVariant=Disabled_SignalSpec  ExternalSaturationOutDataTypeStr=Inherit: Same as second input
  Product : Product
  Pulse Generator : DiscretePulseGenerator  PulseType=Time based  Period=80  PulseWidth=50  PhaseDelay=50
  Saturation 6V1 : Saturate  UpperLimit=5  LowerLimit=-5
  Saturation 6V2 : Saturate  UpperLimit=5  LowerLimit=-5
  Saturation 6V3 : Saturate  UpperLimit=5  LowerLimit=-5
  Scope{,1..3} (4 alike) : Scope
  Sine Wave : Sin  Frequency=0.05  SampleTime=0
  Step : Step  Time=0  SampleTime=0
  Sum : Sum  Inputs=|+-
  Sum1 : Sum  Inputs=|+-
  magTorqueMatrix : Outport
  momentoDipolar : Outport  Port=2
  wires:
  PID Controller3/1 -> Manual Switch1/2
  Saturation 6V1/1 -> Scope1/1, MATLAB Function/2(voltageX), Momento Dipolar X/1  "PWR_mgt X"
  T_deseado/1 -> Sum/1, PID Controller2/1, Sum1/1
  Product/1 -> MATLAB Function/1(B), Cross Product2/2, Cross Product1/2, Cross Product/2
  Manual Switch/1 -> Saturation 6V2/1
  PID Controller1/1 -> Manual Switch/1
  Constant/1 -> Manual Switch2/2, MATLAB Function/4(voltageZ), Manual Switch/2
  Constant1/1 -> Manual Switch1/1
  Manual Switch1/1 -> Saturation 6V1/1
  Momento Dipolar X/1 -> Add1/1, Mgt_ejeX/1
  Mgt_ejeX/1 -> Cross Product/1
  Cross Product/1 -> Goto/1, Add/1, Contribucion de cada Mgt/1  "MgtX"
  Saturation 6V2/1 -> Scope2/1, MATLAB Function/3(voltageY), Momento Dipolar Y/1  "PWR_mgt Y"
  Momento Dipolar Y/1 -> Add1/2, Mgt_ejeY/1
  Mgt_ejeY/1 -> Cross Product1/1
  Cross Product1/1 -> [B], Contribucion de cada Mgt/2, Add/2  "MgtY"
  Add/1 -> Contribucion de cada Mgt1/1, Scope/1, magTorqueMatrix/1
  MATLAB Function/1(magTorqueMatrix) -> Contribucion de cada Mgt1/2
  Add1/1 -> Contribucion de cada Mgt2/1, momentoDipolar/1
  MATLAB Function/2(momentoDipolar) -> Contribucion de cada Mgt2/2
  Manual Switch2/1 -> Saturation 6V3/1
  PID Controller2/1 -> Manual Switch2/1
  Saturation 6V3/1 -> Momento Dipolar Z/1  "PWR_mgt Y"
  Momento Dipolar Z/1 -> Mgt_ejeZ/1
  Mgt_ejeZ/1 -> Cross Product2/1
  Cross Product2/1 -> Add/3  "MgtZ"
  Geomagnetic/1 -> Product/1
  Step/1 -> Product/2
  Sum/1 -> Scope3/1, PID Controller3/1
  Sum1/1 -> PID Controller1/1
  From/1 -> Sum/2
  [B] -> Sum1/2

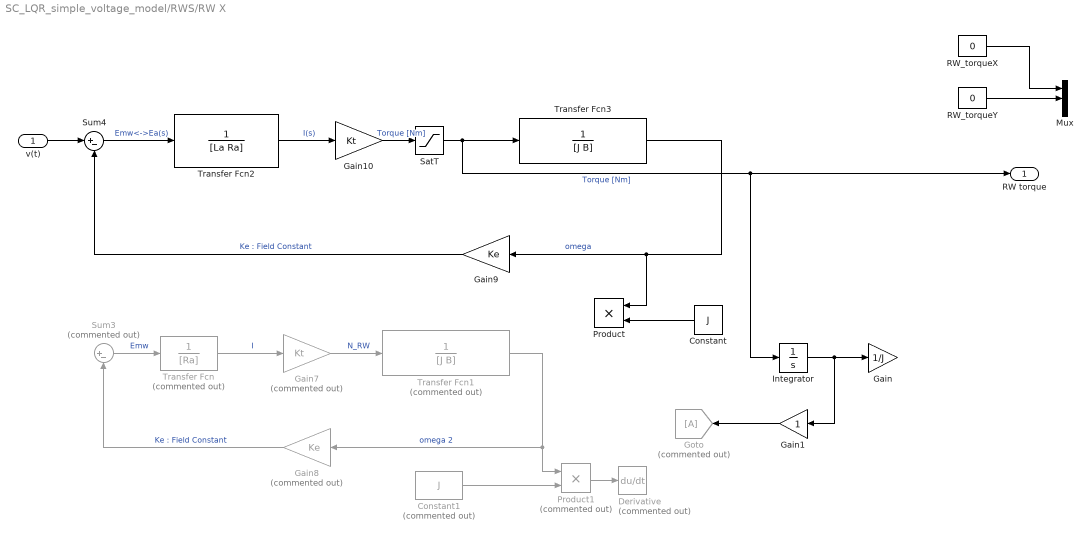
== system SC_LQR_simple_voltage_model/RWS/RW X ==
  v(t) : Inport
  Constant : Constant  Value=J
  Constant1 : Constant  Commented=on  Value=J
  Derivative : Derivative  Commented=on
  Gain : Gain  Gain=1/J
  Gain1 : Gain
  Gain10 : Gain  Gain=Kt
  Gain7 : Gain  Commented=on  Gain=Kt
  Gain8 : Gain  Commented=on  Gain=Ke
  Gain9 : Gain  Gain=Ke
  Goto : Goto  Commented=on
  Integrator : Integrator
  Mux : Mux  Inputs=3
  Product : Product
  Product1 : Product  Commented=on
  RW_torqueX : Constant  Value=0
  RW_torqueY : Constant  Value=0
  SatT : Saturate  UpperLimit=T_max  LowerLimit=-T_max
  Sum3 : Sum  Commented=on  Inputs=|+-
  Sum4 : Sum  Inputs=|+-
  Transfer Fcn : TransferFcn  Commented=on  Denominator=[Ra]
  Transfer Fcn1 : TransferFcn  Commented=on  Denominator=[J B]
  Transfer Fcn2 : TransferFcn  Denominator=[La Ra]
  Transfer Fcn3 : TransferFcn  Denominator=[J B]
  RW torque : Outport  VectorParamsAs1DForOutWhenUnconnected=off
  wires:
  Transfer Fcn2/1 -> Gain10/1  "I(s)"
  Sum4/1 -> Transfer Fcn2/1  "Emw<->Ea(s)"
  Gain9/1 -> Sum4/2  "Ke : Field Constant"
  Transfer Fcn3/1 -> Gain9/1, Product/1  "omega"
  Constant/1 -> Product/2
  Integrator/1 -> Gain1/1, Gain/1
  v(t)/1 -> Sum4/1
  Product1/1 -> Derivative/1
  Constant1/1 -> Product1/2
  Transfer Fcn1/1 -> Product1/1, Gain8/1  "omega 2"
  Gain7/1 -> Transfer Fcn1/1  "N_RW"
  Sum3/1 -> Transfer Fcn/1  "Emw"
  Transfer Fcn/1 -> Gain7/1  "I"
  Gain8/1 -> Sum3/2  "Ke : Field Constant"
  RW_torqueX/1 -> Mux/1
  RW_torqueY/1 -> Mux/2
  Gain10/1 -> SatT/1  "Torque [Nm]"
  Gain1/1 -> Goto/1
  SatT/1 -> RW torque/1, Integrator/1, Transfer Fcn3/1  "Torque [Nm]"

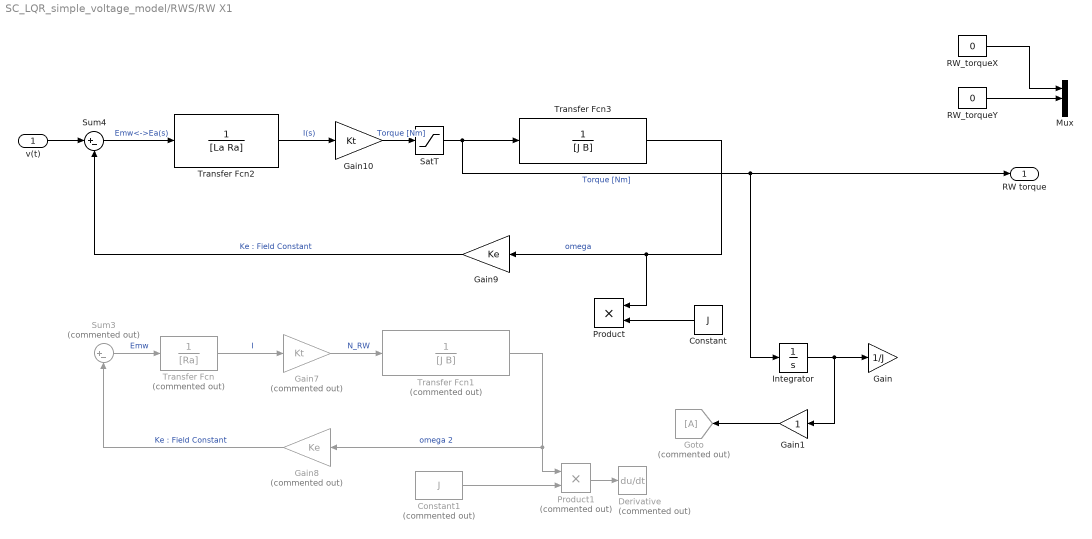
== system SC_LQR_simple_voltage_model/RWS/RW X1 ==
  v(t) : Inport
  Constant : Constant  Value=J
  Constant1 : Constant  Commented=on  Value=J
  Derivative : Derivative  Commented=on
  Gain : Gain  Gain=1/J
  Gain1 : Gain
  Gain10 : Gain  Gain=Kt
  Gain7 : Gain  Commented=on  Gain=Kt
  Gain8 : Gain  Commented=on  Gain=Ke
  Gain9 : Gain  Gain=Ke
  Goto : Goto  Commented=on
  Integrator : Integrator
  Mux : Mux  Inputs=3
  Product : Product
  Product1 : Product  Commented=on
  RW_torqueX : Constant  Value=0
  RW_torqueY : Constant  Value=0
  SatT : Saturate  UpperLimit=T_max  LowerLimit=-T_max
  Sum3 : Sum  Commented=on  Inputs=|+-
  Sum4 : Sum  Inputs=|+-
  Transfer Fcn : TransferFcn  Commented=on  Denominator=[Ra]
  Transfer Fcn1 : TransferFcn  Commented=on  Denominator=[J B]
  Transfer Fcn2 : TransferFcn  Denominator=[La Ra]
  Transfer Fcn3 : TransferFcn  Denominator=[J B]
  RW torque : Outport  VectorParamsAs1DForOutWhenUnconnected=off
  wires:
  SatT/1 -> Transfer Fcn3/1, Integrator/1, RW torque/1  "Torque [Nm]"
  Gain1/1 -> Goto/1
  Gain10/1 -> SatT/1  "Torque [Nm]"
  RW_torqueY/1 -> Mux/2
  RW_torqueX/1 -> Mux/1
  Gain8/1 -> Sum3/2  "Ke : Field Constant"
  Transfer Fcn/1 -> Gain7/1  "I"
  Sum3/1 -> Transfer Fcn/1  "Emw"
  Gain7/1 -> Transfer Fcn1/1  "N_RW"
  Transfer Fcn1/1 -> Gain8/1, Product1/1  "omega 2"
  Constant1/1 -> Product1/2
  Product1/1 -> Derivative/1
  v(t)/1 -> Sum4/1
  Integrator/1 -> Gain/1, Gain1/1
  Constant/1 -> Product/2
  Transfer Fcn3/1 -> Product/1, Gain9/1  "omega"
  Gain9/1 -> Sum4/2  "Ke : Field Constant"
  Sum4/1 -> Transfer Fcn2/1  "Emw<->Ea(s)"
  Transfer Fcn2/1 -> Gain10/1  "I(s)"

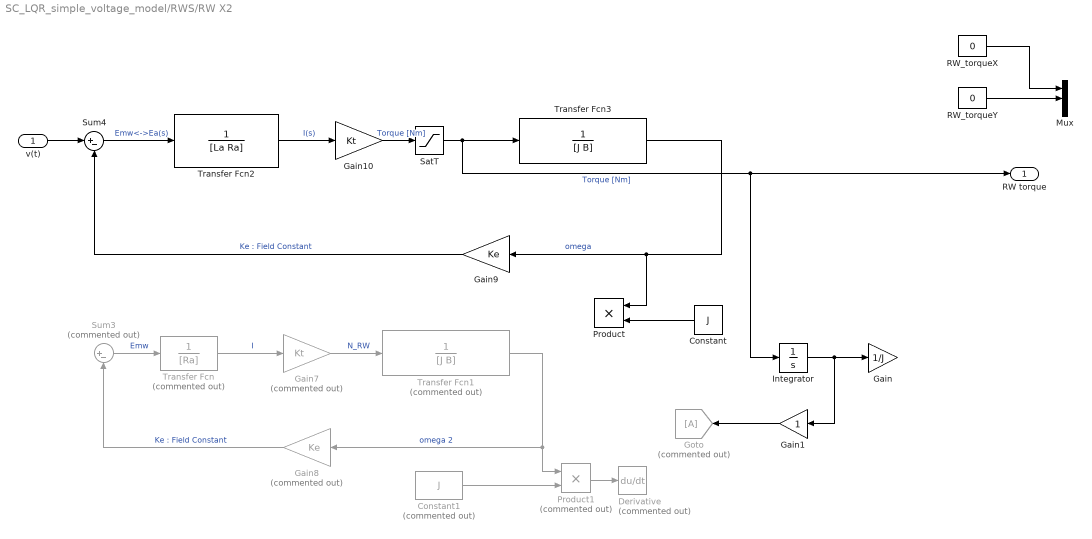
== system SC_LQR_simple_voltage_model/RWS/RW X2 ==
  v(t) : Inport
  Constant : Constant  Value=J
  Constant1 : Constant  Commented=on  Value=J
  Derivative : Derivative  Commented=on
  Gain : Gain  Gain=1/J
  Gain1 : Gain
  Gain10 : Gain  Gain=Kt
  Gain7 : Gain  Commented=on  Gain=Kt
  Gain8 : Gain  Commented=on  Gain=Ke
  Gain9 : Gain  Gain=Ke
  Goto : Goto  Commented=on
  Integrator : Integrator
  Mux : Mux  Inputs=3
  Product : Product
  Product1 : Product  Commented=on
  RW_torqueX : Constant  Value=0
  RW_torqueY : Constant  Value=0
  SatT : Saturate  UpperLimit=T_max  LowerLimit=-T_max
  Sum3 : Sum  Commented=on  Inputs=|+-
  Sum4 : Sum  Inputs=|+-
  Transfer Fcn : TransferFcn  Commented=on  Denominator=[Ra]
  Transfer Fcn1 : TransferFcn  Commented=on  Denominator=[J B]
  Transfer Fcn2 : TransferFcn  Denominator=[La Ra]
  Transfer Fcn3 : TransferFcn  Denominator=[J B]
  RW torque : Outport  VectorParamsAs1DForOutWhenUnconnected=off
  wires:
  Transfer Fcn2/1 -> Gain10/1  "I(s)"
  Sum4/1 -> Transfer Fcn2/1  "Emw<->Ea(s)"
  Gain9/1 -> Sum4/2  "Ke : Field Constant"
  Transfer Fcn3/1 -> Gain9/1, Product/1  "omega"
  Constant/1 -> Product/2
  Integrator/1 -> Gain1/1, Gain/1
  v(t)/1 -> Sum4/1
  Product1/1 -> Derivative/1
  Constant1/1 -> Product1/2
  Transfer Fcn1/1 -> Product1/1, Gain8/1  "omega 2"
  Gain7/1 -> Transfer Fcn1/1  "N_RW"
  Sum3/1 -> Transfer Fcn/1  "Emw"
  Transfer Fcn/1 -> Gain7/1  "I"
  Gain8/1 -> Sum3/2  "Ke : Field Constant"
  RW_torqueX/1 -> Mux/1
  RW_torqueY/1 -> Mux/2
  Gain10/1 -> SatT/1  "Torque [Nm]"
  Gain1/1 -> Goto/1
  SatT/1 -> RW torque/1, Integrator/1, Transfer Fcn3/1  "Torque [Nm]"

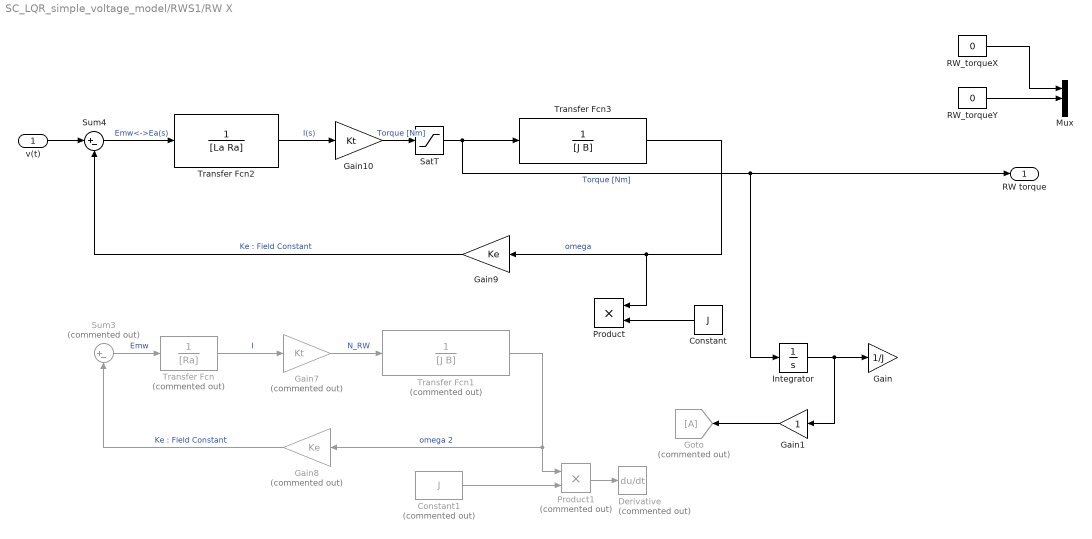
== system SC_LQR_simple_voltage_model/RWS1/RW X ==
  v(t) : Inport
  Constant : Constant  Value=J
  Constant1 : Constant  Commented=on  Value=J
  Derivative : Derivative  Commented=on
  Gain : Gain  Gain=1/J
  Gain1 : Gain
  Gain10 : Gain  Gain=Kt
  Gain7 : Gain  Commented=on  Gain=Kt
  Gain8 : Gain  Commented=on  Gain=Ke
  Gain9 : Gain  Gain=Ke
  Goto : Goto  Commented=on
  Integrator : Integrator
  Mux : Mux  Inputs=3
  Product : Product
  Product1 : Product  Commented=on
  RW_torqueX : Constant  Value=0
  RW_torqueY : Constant  Value=0
  SatT : Saturate  UpperLimit=T_max  LowerLimit=-T_max
  Sum3 : Sum  Commented=on  Inputs=|+-
  Sum4 : Sum  Inputs=|+-
  Transfer Fcn : TransferFcn  Commented=on  Denominator=[Ra]
  Transfer Fcn1 : TransferFcn  Commented=on  Denominator=[J B]
  Transfer Fcn2 : TransferFcn  Denominator=[La Ra]
  Transfer Fcn3 : TransferFcn  Denominator=[J B]
  RW torque : Outport  VectorParamsAs1DForOutWhenUnconnected=off
  wires:
  SatT/1 -> Transfer Fcn3/1, Integrator/1, RW torque/1  "Torque [Nm]"
  Gain1/1 -> Goto/1
  Gain10/1 -> SatT/1  "Torque [Nm]"
  RW_torqueY/1 -> Mux/2
  RW_torqueX/1 -> Mux/1
  Gain8/1 -> Sum3/2  "Ke : Field Constant"
  Transfer Fcn/1 -> Gain7/1  "I"
  Sum3/1 -> Transfer Fcn/1  "Emw"
  Gain7/1 -> Transfer Fcn1/1  "N_RW"
  Transfer Fcn1/1 -> Gain8/1, Product1/1  "omega 2"
  Constant1/1 -> Product1/2
  Product1/1 -> Derivative/1
  v(t)/1 -> Sum4/1
  Integrator/1 -> Gain/1, Gain1/1
  Constant/1 -> Product/2
  Transfer Fcn3/1 -> Product/1, Gain9/1  "omega"
  Gain9/1 -> Sum4/2  "Ke : Field Constant"
  Sum4/1 -> Transfer Fcn2/1  "Emw<->Ea(s)"
  Transfer Fcn2/1 -> Gain10/1  "I(s)"

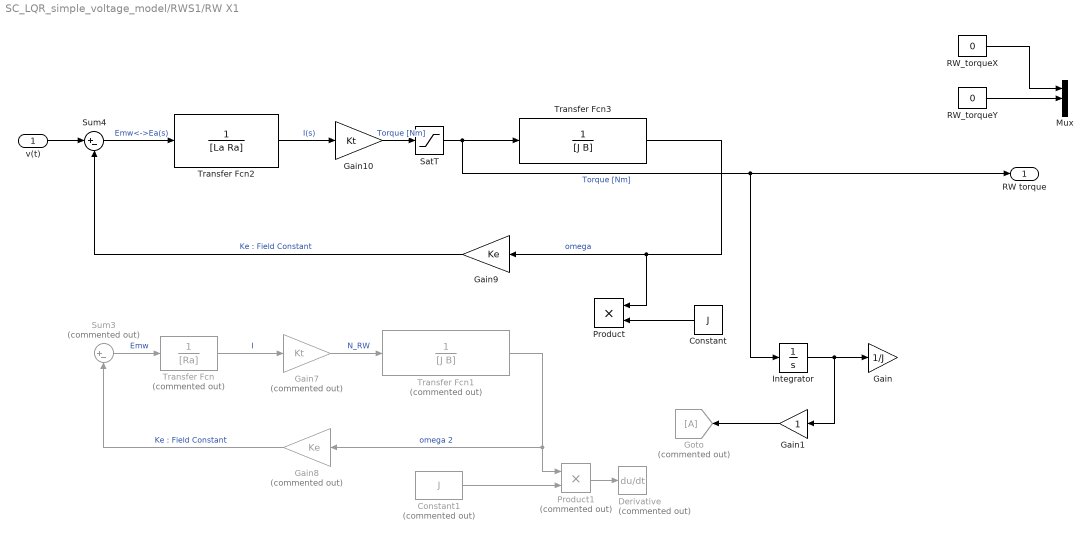
== system SC_LQR_simple_voltage_model/RWS1/RW X1 ==
  v(t) : Inport
  Constant : Constant  Value=J
  Constant1 : Constant  Commented=on  Value=J
  Derivative : Derivative  Commented=on
  Gain : Gain  Gain=1/J
  Gain1 : Gain
  Gain10 : Gain  Gain=Kt
  Gain7 : Gain  Commented=on  Gain=Kt
  Gain8 : Gain  Commented=on  Gain=Ke
  Gain9 : Gain  Gain=Ke
  Goto : Goto  Commented=on
  Integrator : Integrator
  Mux : Mux  Inputs=3
  Product : Product
  Product1 : Product  Commented=on
  RW_torqueX : Constant  Value=0
  RW_torqueY : Constant  Value=0
  SatT : Saturate  UpperLimit=T_max  LowerLimit=-T_max
  Sum3 : Sum  Commented=on  Inputs=|+-
  Sum4 : Sum  Inputs=|+-
  Transfer Fcn : TransferFcn  Commented=on  Denominator=[Ra]
  Transfer Fcn1 : TransferFcn  Commented=on  Denominator=[J B]
  Transfer Fcn2 : TransferFcn  Denominator=[La Ra]
  Transfer Fcn3 : TransferFcn  Denominator=[J B]
  RW torque : Outport  VectorParamsAs1DForOutWhenUnconnected=off
  wires:
  Transfer Fcn2/1 -> Gain10/1  "I(s)"
  Sum4/1 -> Transfer Fcn2/1  "Emw<->Ea(s)"
  Gain9/1 -> Sum4/2  "Ke : Field Constant"
  Transfer Fcn3/1 -> Gain9/1, Product/1  "omega"
  Constant/1 -> Product/2
  Integrator/1 -> Gain1/1, Gain/1
  v(t)/1 -> Sum4/1
  Product1/1 -> Derivative/1
  Constant1/1 -> Product1/2
  Transfer Fcn1/1 -> Product1/1, Gain8/1  "omega 2"
  Gain7/1 -> Transfer Fcn1/1  "N_RW"
  Sum3/1 -> Transfer Fcn/1  "Emw"
  Transfer Fcn/1 -> Gain7/1  "I"
  Gain8/1 -> Sum3/2  "Ke : Field Constant"
  RW_torqueX/1 -> Mux/1
  RW_torqueY/1 -> Mux/2
  Gain10/1 -> SatT/1  "Torque [Nm]"
  Gain1/1 -> Goto/1
  SatT/1 -> RW torque/1, Integrator/1, Transfer Fcn3/1  "Torque [Nm]"
